simulink subsystem "Main"  (R2025b)
settings: Solver=VariableStepAuto  StartTime=0.0  StopTime=10.0  RelTol=1e-3
undefined symbols (not defined in the file): Aero_balance, Aeromaps_ON, air_density, Balance_R_11, Br_coef_of_friction_F, Br_coef_of_friction_R, Br_pistons_area_F, Br_pistons_area_R, CdA, CdA_R_11, ClA, ClA_R_11, CoG_z, Default_Fz_FL, Default_Fz_FR, Default_Fz_RL, Default_Fz_RR, Effective_br_disk_r_F, Effective_br_disk_r_R, Front_brake_balance, Front_brake_pump_area, Front_desired_brake_p_balance, Fx, Fy, Fz, g, Gear_ratio, Iz_wehicle, Iz_wheel, Lf, LLTD, Lock_brake_balance, Lr, Mass, Motor_maximum_power, PRT_efficiency, Rear_brake_pump_area, Roll_Angle_11, SA, SR, start_acc_x, start_acc_y, start_velocity_x, start_velocity_y, start_yaw_acc, start_yaw_rate, Static_Camber_FL, Static_Camber_FR, Static_Camber_RL, Static_Camber_RR, Static_Toe_FL, Static_Toe_FR, Static_Toe_RL, Static_Toe_RR, Steering_Angle_FL, Steering_Angle_FR, Steering_Wheel_Angle, Tire_pressure_FL, Tire_pressure_FR, Tire_pressure_RL ... (+18)
libraries: simulink_extras x9, simulink x7
(part 3 of 3)

== system Main/Powertrain/Motors/Power Limit/Power Calculation ==
  Wheel Speed [rad/s] : Inport
  Motor Torque after TV [Nm] : Inport  Port=2
  Bus Creator : BusCreator  Inputs=4
  Bus Selector : BusSelector  OutputSignals=Motor Torque FL after TV [Nm]
  Bus Selector1 : BusSelector  OutputSignals=Motor Torque FR after TV [Nm]
  Bus Selector2 : BusSelector  OutputSignals=Wheel Speed FL [rad/s]
  Bus Selector3 : BusSelector  OutputSignals=Wheel Speed FR [rad/s]
  Bus Selector4 : BusSelector  OutputSignals=Motor Torque RL after TV [Nm]
  Bus Selector5 : BusSelector  OutputSignals=Wheel Speed RL [rad/s]
  Bus Selector6 : BusSelector  OutputSignals=Motor Torque RR after TV [Nm]
  Bus Selector7 : BusSelector  OutputSignals=Wheel Speed RR [rad/s]
  Gain{,1..3} (4 alike) : Gain  Gain=Gear_ratio
  Product{,1..3} (4 alike) : Product
  Motor Power [W] : Outport
  wires:
  Bus Selector3/1 -> Gain1/1  "<Wheel Speed FR [rad/s]>"
  Gain1/1 -> Product1/2
  Product/1 -> Bus Creator/1  "Motor Power FL [W]"
  Product1/1 -> Bus Creator/2  "Motor Power FR [W]"
  Bus Selector4/1 -> Product2/1  "<Motor Torque RL after TV [Nm]>"
  Bus Selector5/1 -> Gain2/1  "<Wheel Speed RL [rad/s]>"
  Gain2/1 -> Product2/2
  Product2/1 -> Bus Creator/3  "Motor Power RL [W]"
  Bus Selector6/1 -> Product3/1  "<Motor Torque RR after TV [Nm]>"
  Gain3/1 -> Product3/2
  Bus Creator/1 -> Motor Power [W]/1  "Motor Power [W]"
  Bus Selector1/1 -> Product1/1  "<Motor Torque FR after TV [Nm]>"
  Gain/1 -> Product/2
  Bus Selector2/1 -> Gain/1  "<Wheel Speed FL [rad/s]>"
  Product3/1 -> Bus Creator/4  "Motor Power RR [W]"
  Wheel Speed [rad/s]/1 -> Bus Selector2/1, Bus Selector3/1, Bus Selector5/1, Bus Selector7/1
  Bus Selector7/1 -> Gain3/1  "<Wheel Speed RR [rad/s]>"
  Motor Torque after TV [Nm]/1 -> Bus Selector/1, Bus Selector1/1, Bus Selector4/1, Bus Selector6/1
  Bus Selector/1 -> Product/1  "<Motor Torque FL after TV [Nm]>"

== system Main/Powertrain/Motors/Regen Braking/Subsystem ==
  Brake_Preasure_Front : Inport
  Brake_Preasure_Rear : Inport  Port=2
  Desired_Brake_Balance : Inport  Port=3
  Divide2 : Product  Inputs=*/
  Front_Pump_Area : Constant  Value=Front_brake_pump_area
  Product2 : Product
  Product3 : Product
  Product4 : Product
  Rear_Pump_Area : Constant  Value=Rear_brake_pump_area
  Subtract2 : Sum  Inputs=+-
  Sum1 : Sum  Inputs=+-|
  "Motor_Rear_\"Preasure\"" : Outport
  wires:
  Brake_Preasure_Rear/1 -> Subtract2/2
  Subtract2/1 -> "Motor_Rear_\"Preasure\""/1
  Desired_Brake_Balance/1 -> Product2/2, Product3/1
  Front_Pump_Area/1 -> Product4/2
  Sum1/1 -> Divide2/1
  Divide2/1 -> Subtract2/1
  Product2/1 -> Sum1/2
  Product3/1 -> Divide2/2
  Rear_Pump_Area/1 -> Product3/2
  Brake_Preasure_Front/1 -> Product4/1
  Product4/1 -> Product2/1, Sum1/1

== system Main/Powertrain/Motors/Torque Command [Nm]/Switch Case Action Subsystem ==
  APPS : Inport
  Action Port : ActionPort
  1-D Lookup Table1 : Lookup_n-D  NumberOfTableDimensions=1  BreakpointsForDimension1=[0 100]  Table=[0 Torque_limit_max]  InternalRulePriority=Speed  RndMeth=Simplest
  Out1 : Outport
  wires:
  1-D Lookup Table1/1 -> Out1/1
  APPS/1 -> 1-D Lookup Table1/1

== system Main/Powertrain/Motors/Torque Command [Nm]/Switch Case Action Subsystem1 ==
  APPS : Inport
  Action Port : ActionPort
  1-D Lookup Table1 : Lookup_n-D  NumberOfTableDimensions=1  BreakpointsForDimension1=[0 100]  Table=[0 Torque_limit_max]  InternalRulePriority=Speed  RndMeth=Simplest
  Out1 : Outport
  wires:
  APPS/1 -> 1-D Lookup Table1/1
  1-D Lookup Table1/1 -> Out1/1

== system Main/Powertrain/Motors/Torque Command [Nm]/Switch Case Action Subsystem10 ==
  APPS : Inport
  Action Port : ActionPort
  1-D Lookup Table1 : Lookup_n-D  NumberOfTableDimensions=1  BreakpointsForDimension1=[0 100]  Table=[0 Torque_limit_min]  InternalRulePriority=Speed  RndMeth=Simplest
  Out1 : Outport
  wires:
  APPS/1 -> 1-D Lookup Table1/1
  1-D Lookup Table1/1 -> Out1/1

== system Main/Powertrain/Motors/Torque Command [Nm]/Switch Case Action Subsystem2 ==
  APPS : Inport
  Action Port : ActionPort
  1-D Lookup Table1 : Lookup_n-D  NumberOfTableDimensions=1  BreakpointsForDimension1=[0 100]  Table=[0 Torque_limit_9]  InternalRulePriority=Speed  RndMeth=Simplest
  Out1 : Outport
  wires:
  1-D Lookup Table1/1 -> Out1/1
  APPS/1 -> 1-D Lookup Table1/1

== system Main/Powertrain/Motors/Torque Command [Nm]/Switch Case Action Subsystem3 ==
  APPS : Inport
  Action Port : ActionPort
  1-D Lookup Table1 : Lookup_n-D  NumberOfTableDimensions=1  BreakpointsForDimension1=[0 100]  Table=[0 Torque_limit_8]  InternalRulePriority=Speed  RndMeth=Simplest
  Out1 : Outport
  wires:
  APPS/1 -> 1-D Lookup Table1/1
  1-D Lookup Table1/1 -> Out1/1

== system Main/Powertrain/Motors/Torque Command [Nm]/Switch Case Action Subsystem4 ==
  APPS : Inport
  Action Port : ActionPort
  1-D Lookup Table1 : Lookup_n-D  NumberOfTableDimensions=1  BreakpointsForDimension1=[0 100]  Table=[0 Torque_limit_7]  InternalRulePriority=Speed  RndMeth=Simplest
  Out1 : Outport
  wires:
  1-D Lookup Table1/1 -> Out1/1
  APPS/1 -> 1-D Lookup Table1/1

== system Main/Powertrain/Motors/Torque Command [Nm]/Switch Case Action Subsystem5 ==
  APPS : Inport
  Action Port : ActionPort
  1-D Lookup Table1 : Lookup_n-D  NumberOfTableDimensions=1  BreakpointsForDimension1=[0 100]  Table=[0 Torque_limit_6]  InternalRulePriority=Speed  RndMeth=Simplest
  Out1 : Outport
  wires:
  APPS/1 -> 1-D Lookup Table1/1
  1-D Lookup Table1/1 -> Out1/1

== system Main/Powertrain/Motors/Torque Command [Nm]/Switch Case Action Subsystem6 ==
  APPS : Inport
  Action Port : ActionPort
  1-D Lookup Table1 : Lookup_n-D  NumberOfTableDimensions=1  BreakpointsForDimension1=[0 100]  Table=[0 Torque_limit_5]  InternalRulePriority=Speed  RndMeth=Simplest
  Out1 : Outport
  wires:
  APPS/1 -> 1-D Lookup Table1/1
  1-D Lookup Table1/1 -> Out1/1

== system Main/Powertrain/Motors/Torque Command [Nm]/Switch Case Action Subsystem7 ==
  APPS : Inport
  Action Port : ActionPort
  1-D Lookup Table1 : Lookup_n-D  NumberOfTableDimensions=1  BreakpointsForDimension1=[0 100]  Table=[0 Torque_limit_4]  InternalRulePriority=Speed  RndMeth=Simplest
  Out1 : Outport
  wires:
  1-D Lookup Table1/1 -> Out1/1
  APPS/1 -> 1-D Lookup Table1/1

== system Main/Powertrain/Motors/Torque Command [Nm]/Switch Case Action Subsystem8 ==
  APPS : Inport
  Action Port : ActionPort
  1-D Lookup Table1 : Lookup_n-D  NumberOfTableDimensions=1  BreakpointsForDimension1=[0 100]  Table=[0 Torque_limit_3]  InternalRulePriority=Speed  RndMeth=Simplest
  Out1 : Outport
  wires:
  APPS/1 -> 1-D Lookup Table1/1
  1-D Lookup Table1/1 -> Out1/1

== system Main/Powertrain/Motors/Torque Command [Nm]/Switch Case Action Subsystem9 ==
  APPS : Inport
  Action Port : ActionPort
  1-D Lookup Table1 : Lookup_n-D  NumberOfTableDimensions=1  BreakpointsForDimension1=[0 100]  Table=[0 Torque_limit_2]  InternalRulePriority=Speed  RndMeth=Simplest
  Out1 : Outport
  wires:
  1-D Lookup Table1/1 -> Out1/1
  APPS/1 -> 1-D Lookup Table1/1

== system Main/Wheels & Tires/Brakes/Brake_Balance_Adjustment/Enabled Subsystem ==
  In1 : Inport
  Enable : EnablePort
  Out1 : Outport  InitialOutput=[0.5]
  wires:
  In1/1 -> Out1/1

== system Main/Wheels & Tires/Slip Ratio & Slip Angle Calculation/Slip Angle/Slip Angle FL ==
  X Velocity [m/s] : Inport
  Y Velocity [m/s] : Inport  Port=2
  Yaw Rate [rad/s] : Inport  Port=3
  Steering Angle FL [rad] : Inport  Port=4
  Atan : Trigonometry  Operator=atan
  Constant : Constant  Value=Lf
  Constant1 : Constant  Value=Track_Front
  Divide : Product  Inputs=*/
  Gain : Gain  Gain=1/2
  Product : Product
  Product1 : Product
  Subtract : Sum
  Subtract1 : Sum
  Subtract2 : Sum  Inputs=+-
  Slip Angle FL [rad] : Outport
  wires:
  Yaw Rate [rad/s]/1 -> Product1/1, Product/2
  X Velocity [m/s]/1 -> Subtract1/2
  Y Velocity [m/s]/1 -> Subtract/1
  Atan/1 -> Subtract2/1
  Constant/1 -> Product/1
  Subtract2/1 -> Slip Angle FL [rad]/1
  Product1/1 -> Subtract1/1
  Divide/1 -> Atan/1
  Gain/1 -> Product1/2
  Constant1/1 -> Gain/1
  Subtract1/1 -> Divide/2
  Steering Angle FL [rad]/1 -> Subtract2/2
  Product/1 -> Subtract/2
  Subtract/1 -> Divide/1

== system Main/Wheels & Tires/Slip Ratio & Slip Angle Calculation/Slip Angle/Slip Angle FR ==
  X Velocity [m/s] : Inport
  Y Velocity [m/s] : Inport  Port=2
  Yaw Rate [rad/s] : Inport  Port=3
  Steering Angle FR [rad] : Inport  Port=4
  Atan : Trigonometry  Operator=atan
  Constant : Constant  Value=Lf
  Constant1 : Constant  Value=Track_Front
  Divide : Product  Inputs=*/
  Gain : Gain  Gain=1/2
  Product : Product
  Product1 : Product
  Subtract : Sum
  Subtract1 : Sum  Inputs=-+
  Subtract2 : Sum  Inputs=+-
  Slip Angle FR [rad] : Outport
  wires:
  X Velocity [m/s]/1 -> Subtract1/2
  Y Velocity [m/s]/1 -> Subtract/1
  Yaw Rate [rad/s]/1 -> Product1/1, Product/2
  Atan/1 -> Subtract2/1
  Subtract/1 -> Divide/1
  Subtract1/1 -> Divide/2
  Constant1/1 -> Gain/1
  Product/1 -> Subtract/2
  Steering Angle FR [rad]/1 -> Subtract2/2
  Constant/1 -> Product/1
  Gain/1 -> Product1/2
  Divide/1 -> Atan/1
  Product1/1 -> Subtract1/1
  Subtract2/1 -> Slip Angle FR [rad]/1

== system Main/Wheels & Tires/Slip Ratio & Slip Angle Calculation/Slip Angle/Slip Angle RL ==
  X Velocity [m/s] : Inport
  Y Velocity [m/s] : Inport  Port=2
  Yaw Rate [rad/s] : Inport  Port=3
  Steering Angle RL [rad] : Inport  Port=4
  Atan : Trigonometry  Operator=atan
  Constant : Constant  Value=Lr
  Constant1 : Constant  Value=Track_Rear
  Divide : Product  Inputs=*/
  Gain : Gain  Gain=1/2
  Product : Product
  Product1 : Product
  Subtract : Sum  Inputs=+-
  Subtract1 : Sum
  Subtract2 : Sum  Inputs=+-
  Slip Angle RL [rad] : Outport
  wires:
  X Velocity [m/s]/1 -> Subtract1/2
  Y Velocity [m/s]/1 -> Subtract/1
  Yaw Rate [rad/s]/1 -> Product1/1, Product/2
  Atan/1 -> Subtract2/1
  Gain/1 -> Product1/2
  Steering Angle RL [rad]/1 -> Subtract2/2
  Constant1/1 -> Gain/1
  Product/1 -> Subtract/2
  Subtract1/1 -> Divide/2
  Subtract/1 -> Divide/1
  Subtract2/1 -> Slip Angle RL [rad]/1
  Constant/1 -> Product/1
  Product1/1 -> Subtract1/1
  Divide/1 -> Atan/1

== system Main/Wheels & Tires/Slip Ratio & Slip Angle Calculation/Slip Angle/Slip Angle RR ==
  X Velocity [m/s] : Inport
  Y Velocity [m/s] : Inport  Port=2
  Yaw Rate [rad/s] : Inport  Port=3
  Steering Angle RR [rad] : Inport  Port=4
  Atan : Trigonometry  Operator=atan
  Constant : Constant  Value=Lr
  Constant1 : Constant  Value=Track_Rear
  Divide : Product  Inputs=*/
  Gain : Gain  Gain=1/2
  Product : Product
  Product1 : Product
  Subtract : Sum  Inputs=+-
  Subtract1 : Sum  Inputs=-+
  Subtract2 : Sum  Inputs=+-
  Slip Angle RR [rad] : Outport
  wires:
  Yaw Rate [rad/s]/1 -> Product1/1, Product/2
  X Velocity [m/s]/1 -> Subtract1/2
  Y Velocity [m/s]/1 -> Subtract/1
  Atan/1 -> Subtract2/1
  Constant/1 -> Product/1
  Subtract2/1 -> Slip Angle RR [rad]/1
  Product1/1 -> Subtract1/1
  Divide/1 -> Atan/1
  Gain/1 -> Product1/2
  Constant1/1 -> Gain/1
  Subtract1/1 -> Divide/2
  Steering Angle RR [rad]/1 -> Subtract2/2
  Product/1 -> Subtract/2
  Subtract/1 -> Divide/1

== system Main/Wheels & Tires/Slip Ratio & Slip Angle Calculation/Slip Ratio /Slip ratio FL ==
  Wheel Speed FL [rad/s] : Inport
  X Velocity [m/s] : Inport  Port=2
  Yaw Rate [rad/s] : Inport  Port=3
  Constant4 : Constant  Value=Tire_radius
  Divide1 : Product
  Gain : Gain  Gain=Track_Front/2
  Product2 : Product  Inputs=*/
  Saturation1 : Saturate  UpperLimit=1  LowerLimit=-1
  Subtract : Sum  Inputs=+-
  Subtract2 : Sum  Inputs=+-
  Slip Ratio FL : Outport
  wires:
  Yaw Rate [rad/s]/1 -> Gain/1
  Subtract/1 -> Product2/2, Subtract2/2  "Wheel X Velocity FL [m/s]"
  Gain/1 -> Subtract/2
  X Velocity [m/s]/1 -> Subtract/1
  Saturation1/1 -> Slip Ratio FL/1
  Wheel Speed FL [rad/s]/1 -> Divide1/2
  Constant4/1 -> Divide1/1
  Subtract2/1 -> Product2/1
  Product2/1 -> Saturation1/1
  Divide1/1 -> Subtract2/1

== system Main/Wheels & Tires/Slip Ratio & Slip Angle Calculation/Slip Ratio /Slip ratio FR ==
  Wheel Speed FR [rad/s] : Inport
  X Velocity [m/s] : Inport  Port=2
  Yaw Rate [rad/s] : Inport  Port=3
  Constant4 : Constant  Value=Tire_radius
  Divide1 : Product
  Gain : Gain  Gain=Track_Front/2
  Product2 : Product  Inputs=*/
  Saturation1 : Saturate  UpperLimit=1  LowerLimit=-1
  Subtract : Sum  Inputs=+-
  Subtract2 : Sum  Inputs=+-
  Slip Ratio FR : Outport
  wires:
  Yaw Rate [rad/s]/1 -> Gain/1
  Divide1/1 -> Subtract2/1
  Subtract/1 -> Product2/2, Subtract2/2  "Wheel X Velocity FR [m/s]"
  Wheel Speed FR [rad/s]/1 -> Divide1/2
  Product2/1 -> Saturation1/1
  Gain/1 -> Subtract/2
  X Velocity [m/s]/1 -> Subtract/1
  Subtract2/1 -> Product2/1
  Constant4/1 -> Divide1/1
  Saturation1/1 -> Slip Ratio FR/1

== system Main/Wheels & Tires/Slip Ratio & Slip Angle Calculation/Slip Ratio /Slip ratio RL ==
  Wheel Speed RL [rad/s] : Inport
  X Velocity [m/s] : Inport  Port=2
  Yaw Rate [rad/s] : Inport  Port=3
  Constant4 : Constant  Value=Tire_radius
  Divide : Product
  Gain : Gain  Gain=Track_Rear/2
  Max : MinMax  Function=max  Inputs=2
  Product2 : Product  Inputs=*/
  Saturation2 : Saturate  UpperLimit=1  LowerLimit=-1
  Subtract : Sum  Inputs=+-
  Subtract2 : Sum  Inputs=+-
  Slip Ratio RL : Outport
  wires:
  Yaw Rate [rad/s]/1 -> Gain/1
  Subtract/1 -> Max/2, Subtract2/2  "Wheel X Velocity RL [m/s]"
  Gain/1 -> Subtract/2
  Saturation2/1 -> Slip Ratio RL/1
  Constant4/1 -> Divide/1
  Max/1 -> Product2/2
  Wheel Speed RL [rad/s]/1 -> Divide/2
  Product2/1 -> Saturation2/1
  Divide/1 -> Subtract2/1, Max/1
  X Velocity [m/s]/1 -> Subtract/1
  Subtract2/1 -> Product2/1

== system Main/Wheels & Tires/Slip Ratio & Slip Angle Calculation/Slip Ratio /Slip ratio RR ==
  Wheel Speed RR [rad/s] : Inport
  X Velocity [m/s] : Inport  Port=2
  Yaw Rate [rad/s] : Inport  Port=3
  Constant4 : Constant  Value=Tire_radius
  Divide : Product
  Gain : Gain  Gain=Track_Rear/2
  Max : MinMax  Function=max  Inputs=2
  Product2 : Product  Inputs=*/
  Saturation2 : Saturate  UpperLimit=1  LowerLimit=-1
  Subtract : Sum  Inputs=+-
  Subtract2 : Sum  Inputs=+-
  Slip Ratio RR : Outport
  wires:
  Yaw Rate [rad/s]/1 -> Gain/1
  Saturation2/1 -> Slip Ratio RR/1
  Max/1 -> Product2/2
  Subtract2/1 -> Product2/1
  Wheel Speed RR [rad/s]/1 -> Divide/2
  Gain/1 -> Subtract/2
  Constant4/1 -> Divide/1
  Divide/1 -> Subtract2/1, Max/1
  Subtract/1 -> Max/2, Subtract2/2  "Wheel X Velocity RR [m/s]"
  Product2/1 -> Saturation2/1
  X Velocity [m/s]/1 -> Subtract/1

== matlab function Main/Wheels & Tires/Mz/Pure Mz/Pure Mz FR ==
  settings: updateMethod=DISCRETE
  data: pressure input; gamma input; Fz input; alpha input; Mz0 output
function Mz0 = PureMz(pressure, gamma, Fz, alpha)

persistent CoeffLat SFLat CoeffAlign SFAlign

if isempty(CoeffLat) || isempty(SFLat)

    mf = load('mfparams_2.mat'); 
    mfparams = mf.mfparams;
    

    CoeffLat = Tire_Coefficients(mfparams, 'c_lat'); 
    SFLat = Tire_Scaling_Factors(mfparams, 'sf_lat');

    CoeffAlign = Tire_Coefficients(mfparams, 'c_align'); 
    SFAlign = Tire_Scaling_Factors(mfparams, 'sf_align');
end

Mz0 = AligningMF(CoeffAlign,SFAlign,alpha,Fz,gamma, pressure, CoeffLat,SFLat);

end

== matlab function Main/Wheels & Tires/Mz/Pure Mz/Pure Mz FL ==
  settings: updateMethod=DISCRETE
  data: pressure input; gamma input; Fz input; alpha input; Mz0 output
function Mz0 = PureMz(pressure, gamma, Fz, alpha)

persistent CoeffLat SFLat CoeffAlign SFAlign

if isempty(CoeffLat) || isempty(SFLat)

    mf = load('mfparams_2.mat'); 
    mfparams = mf.mfparams;
    

    CoeffLat = Tire_Coefficients(mfparams, 'c_lat'); 
    SFLat = Tire_Scaling_Factors(mfparams, 'sf_lat');

    CoeffAlign = Tire_Coefficients(mfparams, 'c_align'); 
    SFAlign = Tire_Scaling_Factors(mfparams, 'sf_align');
end

Mz0 = AligningMF(CoeffAlign,SFAlign,alpha,Fz,gamma, pressure, CoeffLat,SFLat);

end

== matlab function Main/Wheels & Tires/Fx/Combined Fx/Combined Fx FL ==
  settings: updateMethod=DISCRETE
  data: pressure input; gamma input; Fz input; kappa input; Fx output; alpha input
function Fx = CombinedFx(pressure, gamma, Fz, kappa, alpha)

persistent CoeffLong SFLong

if isempty(CoeffLong) || isempty(SFLong)

    mf = load('mfparams_2.mat'); 
    mfparams = mf.mfparams;
    
    CoeffLong = Tire_Coefficients(mfparams, 'c_long');
    SFLong = Tire_Scaling_Factors(mfparams, 'sf_long');
end

Fx = CombinedLongitudinalMF(CoeffLong,SFLong,kappa,alpha,Fz,gamma,pressure);

end

== matlab function Main/Wheels & Tires/Fy/Pure Fy NEW/Pure Fy FR ==
  settings: updateMethod=DISCRETE
  data: pressure input; gamma input; Fz input; alpha input; Fy0 output
function Fy0 = PureFy(pressure, gamma, Fz, alpha)

persistent CoeffLat SFLat

if isempty(CoeffLat) || isempty(SFLat)
    mf = load('mfparams_2.mat'); 
    mfparams = mf.mfparams;
    
    CoeffLat = Tire_Coefficients(mfparams, 'c_lat');
    SFLat = Tire_Scaling_Factors(mfparams, 'sf_lat');
end

Fy0 = LateralMF(CoeffLat, SFLat, alpha, Fz, gamma, pressure);

end

== matlab function Main/Wheels & Tires/Mz/Pure Mz/Pure Mz RR ==
  settings: updateMethod=DISCRETE
  data: pressure input; gamma input; Fz input; alpha input; Mz0 output
function Mz0 = PureMz(pressure, gamma, Fz, alpha)

persistent CoeffLat SFLat CoeffAlign SFAlign

if isempty(CoeffLat) || isempty(SFLat)

    mf = load('mfparams_2.mat'); 
    mfparams = mf.mfparams;
    

    CoeffLat = Tire_Coefficients(mfparams, 'c_lat'); 
    SFLat = Tire_Scaling_Factors(mfparams, 'sf_lat');

    CoeffAlign = Tire_Coefficients(mfparams, 'c_align'); 
    SFAlign = Tire_Scaling_Factors(mfparams, 'sf_align');
end

Mz0 = AligningMF(CoeffAlign,SFAlign,alpha,Fz,gamma, pressure, CoeffLat,SFLat);

end

== matlab function Main/Wheels & Tires/Fx/Combined Fx/Combined Fx FR ==
  settings: updateMethod=DISCRETE
  data: pressure input; gamma input; Fz input; kappa input; Fx output; alpha input
function Fx = CombinedFx(pressure, gamma, Fz, kappa, alpha)

persistent CoeffLong SFLong

if isempty(CoeffLong) || isempty(SFLong)

    mf = load('mfparams_2.mat'); 
    mfparams = mf.mfparams;
    
    CoeffLong = Tire_Coefficients(mfparams, 'c_long');
    SFLong = Tire_Scaling_Factors(mfparams, 'sf_long');
end

Fx = CombinedLongitudinalMF(CoeffLong,SFLong,kappa,alpha,Fz,gamma,pressure);

end

== matlab function Main/Wheels & Tires/Fx/Combined Fx/Combined Fx RL ==
  settings: updateMethod=DISCRETE
  data: pressure input; gamma input; Fz input; kappa input; Fx output; alpha input
function Fx = CombinedFx(pressure, gamma, Fz, kappa, alpha)

persistent CoeffLong SFLong

if isempty(CoeffLong) || isempty(SFLong)

    mf = load('mfparams_2.mat'); 
    mfparams = mf.mfparams;
    
    CoeffLong = Tire_Coefficients(mfparams, 'c_long');
    SFLong = Tire_Scaling_Factors(mfparams, 'sf_long');
end

Fx = CombinedLongitudinalMF(CoeffLong,SFLong,kappa,alpha,Fz,gamma,pressure);

end

== matlab function Main/Wheels & Tires/Fx/Combined Fx/Combined Fx RR ==
  settings: updateMethod=DISCRETE
  data: pressure input; gamma input; Fz input; kappa input; Fx output; alpha input
function Fx = CombinedFx(pressure, gamma, Fz, kappa, alpha)

persistent CoeffLong SFLong

if isempty(CoeffLong) || isempty(SFLong)

    mf = load('mfparams_2.mat'); 
    mfparams = mf.mfparams;
    
    CoeffLong = Tire_Coefficients(mfparams, 'c_long');
    SFLong = Tire_Scaling_Factors(mfparams, 'sf_long');
end

Fx = CombinedLongitudinalMF(CoeffLong,SFLong,kappa,alpha,Fz,gamma,pressure);

end

== matlab function Main/Wheels & Tires/Fy/Combined Fy/Combined Fy FR ==
  settings: updateMethod=DISCRETE
  data: pressure input; gamma input; Fz input; alpha input; kappa input; Fy output
function Fy = CombinedFy(pressure, gamma, Fz, alpha, kappa)

persistent CoeffLat SFLat

if isempty(CoeffLat) || isempty(SFLat)
    % Load only once
    mf = load('mfparams_2.mat'); 
    mfparams = mf.mfparams;
    
    CoeffLat = Tire_Coefficients(mfparams, 'c_lat');
    SFLat = Tire_Scaling_Factors(mfparams, 'sf_lat');
end

Fy = CombinedLateralMF(CoeffLat, SFLat, kappa, alpha, Fz, gamma, pressure);

end

== matlab function Main/Wheels & Tires/Fy/Combined Fy/Combined Fy RL ==
  settings: updateMethod=DISCRETE
  data: pressure input; gamma input; Fz input; alpha input; kappa input; Fy output
function Fy = CombinedFy(pressure, gamma, Fz, alpha, kappa)

persistent CoeffLat SFLat

if isempty(CoeffLat) || isempty(SFLat)
    % Load only once
    mf = load('mfparams_2.mat'); 
    mfparams = mf.mfparams;
    
    CoeffLat = Tire_Coefficients(mfparams, 'c_lat');
    SFLat = Tire_Scaling_Factors(mfparams, 'sf_lat');
end

Fy = CombinedLateralMF(CoeffLat, SFLat, kappa, alpha, Fz, gamma, pressure);

end

== matlab function Main/Wheels & Tires/Fy/Combined Fy/Combined Fy RR ==
  settings: updateMethod=DISCRETE
  data: pressure input; gamma input; Fz input; alpha input; kappa input; Fy output
function Fy = CombinedFy(pressure, gamma, Fz, alpha, kappa)

persistent CoeffLat SFLat

if isempty(CoeffLat) || isempty(SFLat)
    % Load only once
    mf = load('mfparams_2.mat'); 
    mfparams = mf.mfparams;
    
    CoeffLat = Tire_Coefficients(mfparams, 'c_lat');
    SFLat = Tire_Scaling_Factors(mfparams, 'sf_lat');
end

Fy = CombinedLateralMF(CoeffLat, SFLat, kappa, alpha, Fz, gamma, pressure);

end

== matlab function Main/Wheels & Tires/Fy/Combined Fy/Combined Fy FL ==
  settings: updateMethod=DISCRETE
  data: pressure input; gamma input; Fz input; alpha input; kappa input; Fy output
function Fy = CombinedFy(pressure, gamma, Fz, alpha, kappa)

persistent CoeffLat SFLat

if isempty(CoeffLat) || isempty(SFLat)
    % Load only once
    mf = load('mfparams_2.mat'); 
    mfparams = mf.mfparams;
    
    CoeffLat = Tire_Coefficients(mfparams, 'c_lat');
    SFLat = Tire_Scaling_Factors(mfparams, 'sf_lat');
end

Fy = CombinedLateralMF(CoeffLat, SFLat, kappa, alpha, Fz, gamma, pressure);

end



function Fy0 = PureFy(pressure, gamma, Fz, alpha)

persistent CoeffLat SFLat

if isempty(CoeffLat) || isempty(SFLat)
    mf = load('mfparams_2.mat'); 
    mfparams = mf.mfparams;
    
    CoeffLat = Tire_Coefficients(mfparams, 'c_lat');
    SFLat = Tire_Scaling_Factors(mfparams, 'sf_lat');
end

Fy0 = LateralMF(CoeffLat, SFLat, alpha, Fz, gamma, pressure);

end

== matlab function Main/Wheels & Tires/Fy/Pure Fy NEW/Pure Fy FL ==
  settings: updateMethod=DISCRETE
  data: pressure input; gamma input; Fz input; alpha input; Fy0 output
function Fy0 = PureFy(pressure, gamma, Fz, alpha)

persistent CoeffLat SFLat

if isempty(CoeffLat) || isempty(SFLat)
    mf = load('mfparams_2.mat'); 
    mfparams = mf.mfparams;
    
    CoeffLat = Tire_Coefficients(mfparams, 'c_lat');
    SFLat = Tire_Scaling_Factors(mfparams, 'sf_lat');
end

Fy0 = LateralMF(CoeffLat, SFLat, alpha, Fz, gamma, pressure);

end

== matlab function Main/Wheels & Tires/Fy/Pure Fy NEW/Pure Fy RL ==
  settings: updateMethod=DISCRETE
  data: pressure input; gamma input; Fz input; alpha input; Fy0 output
function Fy0 = PureFy(pressure, gamma, Fz, alpha)

persistent CoeffLat SFLat

if isempty(CoeffLat) || isempty(SFLat)
    mf = load('mfparams_2.mat'); 
    mfparams = mf.mfparams;
    
    CoeffLat = Tire_Coefficients(mfparams, 'c_lat');
    SFLat = Tire_Scaling_Factors(mfparams, 'sf_lat');
end

Fy0 = LateralMF(CoeffLat, SFLat, alpha, Fz, gamma, pressure);

end

== matlab function Main/Wheels & Tires/Fy/Pure Fy NEW/Pure Fy RR ==
  settings: updateMethod=DISCRETE
  data: pressure input; gamma input; Fz input; alpha input; Fy0 output
function Fy0 = PureFy(pressure, gamma, Fz, alpha)

persistent CoeffLat SFLat

if isempty(CoeffLat) || isempty(SFLat)
    mf = load('mfparams_2.mat'); 
    mfparams = mf.mfparams;
    
    CoeffLat = Tire_Coefficients(mfparams, 'c_lat');
    SFLat = Tire_Scaling_Factors(mfparams, 'sf_lat');
end

Fy0 = LateralMF(CoeffLat, SFLat, alpha, Fz, gamma, pressure);

end

== matlab function Main/Wheels & Tires/Fx/Pure Fx NEW/Pure Fx FL ==
  settings: updateMethod=DISCRETE
  data: pressure input; gamma input; Fz input; kappa input; Fx0 output
function Fx0 = PureFx(pressure, gamma, Fz, kappa)

persistent CoeffLong SFLat

if isempty(CoeffLong) || isempty(SFLat)

    mf = load('mfparams_2.mat'); 
    mfparams = mf.mfparams;
    
    CoeffLong = Tire_Coefficients(mfparams, 'c_long');
    SFLat = Tire_Scaling_Factors(mfparams, 'sf_long');
end

Fx0 = LongitudinalMF(CoeffLong, SFLat, kappa, Fz, gamma, pressure);

end

== matlab function Main/Wheels & Tires/Fx/Pure Fx NEW/Pure Fx FR ==
  settings: updateMethod=DISCRETE
  data: pressure input; gamma input; Fz input; kappa input; Fx0 output
function Fx0 = PureFx(pressure, gamma, Fz, kappa)

persistent CoeffLong SFLat

if isempty(CoeffLong) || isempty(SFLat)

    mf = load('mfparams_2.mat'); 
    mfparams = mf.mfparams;
    
    CoeffLong = Tire_Coefficients(mfparams, 'c_long');
    SFLat = Tire_Scaling_Factors(mfparams, 'sf_long');
end

Fx0 = LongitudinalMF(CoeffLong, SFLat, kappa, Fz, gamma, pressure);

end

== matlab function Main/Wheels & Tires/Fx/Pure Fx NEW/Pure Fx RL ==
  settings: updateMethod=DISCRETE
  data: pressure input; gamma input; Fz input; kappa input; Fx0 output
function Fx0 = PureFx(pressure, gamma, Fz, kappa)

persistent CoeffLong SFLat

if isempty(CoeffLong) || isempty(SFLat)

    mf = load('mfparams_2.mat'); 
    mfparams = mf.mfparams;
    
    CoeffLong = Tire_Coefficients(mfparams, 'c_long');
    SFLat = Tire_Scaling_Factors(mfparams, 'sf_long');
end

Fx0 = LongitudinalMF(CoeffLong, SFLat, kappa, Fz, gamma, pressure);

end

== matlab function Main/Wheels & Tires/Fx/Pure Fx NEW/Pure Fx RR ==
  settings: updateMethod=DISCRETE
  data: pressure input; gamma input; Fz input; kappa input; Fx0 output
function Fx0 = PureFx(pressure, gamma, Fz, kappa)

persistent CoeffLong SFLat

if isempty(CoeffLong) || isempty(SFLat)

    mf = load('mfparams_2.mat'); 
    mfparams = mf.mfparams;
    
    CoeffLong = Tire_Coefficients(mfparams, 'c_long');
    SFLat = Tire_Scaling_Factors(mfparams, 'sf_long');
end

Fx0 = LongitudinalMF(CoeffLong, SFLat, kappa, Fz, gamma, pressure);

end

== matlab function Main/Wheels & Tires/Mz/Pure Mz/Pure Mz RL ==
  settings: updateMethod=DISCRETE
  data: pressure input; gamma input; Fz input; alpha input; Mz0 output
function Mz0 = PureMz(pressure, gamma, Fz, alpha)

persistent CoeffLat SFLat CoeffAlign SFAlign

if isempty(CoeffLat) || isempty(SFLat)

    mf = load('mfparams_2.mat'); 
    mfparams = mf.mfparams;
    

    CoeffLat = Tire_Coefficients(mfparams, 'c_lat'); 
    SFLat = Tire_Scaling_Factors(mfparams, 'sf_lat');

    CoeffAlign = Tire_Coefficients(mfparams, 'c_align'); 
    SFAlign = Tire_Scaling_Factors(mfparams, 'sf_align');
end

Mz0 = AligningMF(CoeffAlign,SFAlign,alpha,Fz,gamma, pressure, CoeffLat,SFLat);

end
